simulink model "TP1_Simulink"  (R2021a)
settings: Solver=VariableStepAuto  StartTime=0.0  StopTime=3000  RelTol=1e-3
values from neighbouring files (symbols this model uses):
  A_sim = double(subs(As,{x,u},{x_e,u_e}))    [TPI_Matlab.m]    (also in tp1.m)
  B_sim = double(subs(Bs,{x,u},{x_e,u_e}))    [TPI_Matlab.m]    (also in tp1.m)
  C_sim = double(subs(Cs,{x,u},{x_e,u_e}))    [TPI_Matlab.m]    (also in tp1.m)
  D_sim = double(subs(Ds,{x,u},{x_e,u_e}))    [TPI_Matlab.m]    (also in tp1.m)
  h_e = 0.45    [TPI_Matlab.m]    (also in tp1.m)
  Q_i = 8e-3/60    (= 0.000133333333333)    [TPI_Matlab.m]    (also in ej1.m; tp1.m)
  u_e = Q_i/(pi * d^2 * sqrt(2*G*x_e)/4)    [TPI_Matlab.m]    (also in ej1.m = Q_i./(pi * d^2 * sqrt(2*G*x_e)/4); tp1.m)
  x_e = 0.45    [TPI_Matlab.m]    (also in ej1.m = (0.1:0.1:0.8); tp1.m)
libraries: cstblocks x4
settings Model: Creator=Cristian  LastModifiedBy=nnobi

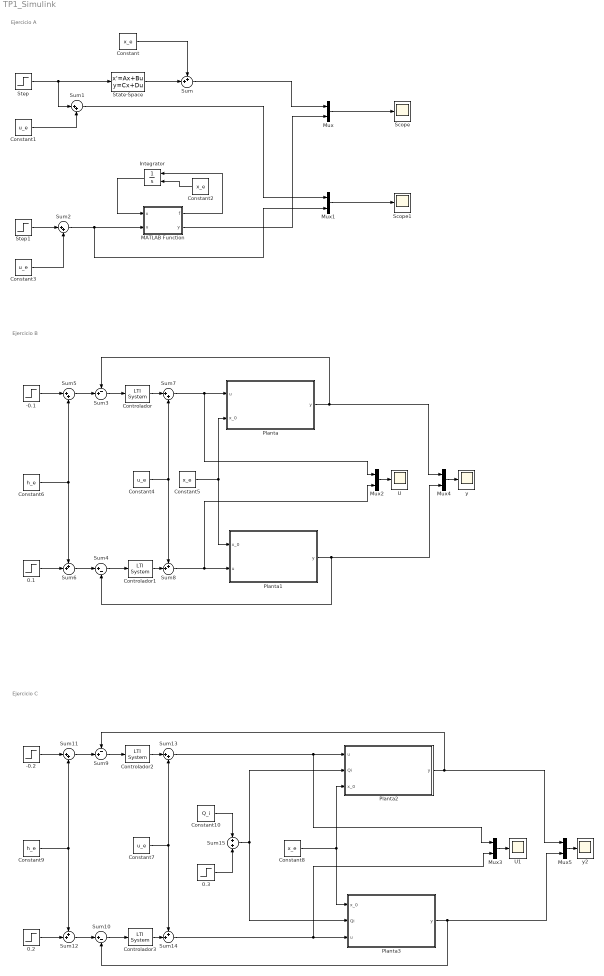
== system TP1_Simulink ==
  note: Ejercicio B
  note: Ejercicio A
  note: Ejercicio C
  -0.1 : Step  Time=60  After=-0.1  SampleTime=0
  -0.2 : Step  Time=60  After=-0.1  SampleTime=0
  0.1 : Step  Time=60  After=0.1  SampleTime=0
  0.2 : Step  Time=60  After=0.1  SampleTime=0
  0.3 : Step  Time=1000  After=-0.1*Q_i  SampleTime=0
  Constant{,2,5,8} (4 alike) : Constant  Value=x_e
  Constant{1,3..4,7} (4 alike) : Constant  Value=u_e
  Constant10 : Constant  Value=Q_i
  Constant6 : Constant  Value=h_e
  Constant9 : Constant  Value=h_e
  Controlador{,1..3} (4 alike) : cstblocks/LTI System  sys=C  IC=[]
  Integrator : Integrator  InitialConditionSource=external
  MATLAB Function : MATLAB Function  TreatAsAtomicUnit=on
  Mux{,1..5} (6 alike) : Mux  Inputs=2
  Planta : Subsystem
  Planta1 : Subsystem
  Planta2 : Subsystem
  Planta3 : Subsystem
  Scope : Scope
  Scope1 : Scope
  State-Space : StateSpace  A=A_sim  B=B_sim  C=C_sim  D=D_sim  InitialCondition=0
  Step : Step  Time=60  After=0.1*u_e  SampleTime=0
  Step1 : Step  Time=60  After=0.1*u_e  SampleTime=0
  Sum{,6,8,12,14} (5 alike) : Sum  Inputs=++|
  Sum{1..2,5,7,11,13} (6 alike) : Sum  Inputs=|++
  Sum10 : Sum  Inputs=|+-
  Sum15 : Sum
  Sum3 : Sum  Inputs=-+|
  Sum4 : Sum  Inputs=|+-
  Sum9 : Sum  Inputs=-+|
  U : Scope
  U1 : Scope
  y : Scope
  y2 : Scope
  wires:
  Step/1 -> Sum1/1, State-Space/1
  State-Space/1 -> Sum/2
  Constant/1 -> Sum/1
  Constant1/1 -> Sum1/2
  Step1/1 -> Sum2/1
  Constant3/1 -> Sum2/2
  Constant2/1 -> Integrator/2
  Sum2/1 -> Mux1/2, MATLAB Function/2(u)
  Integrator/1 -> MATLAB Function/1(x)
  MATLAB Function/1(f) -> Integrator/1
  Mux/1 -> Scope/1
  Sum/1 -> Mux/1
  MATLAB Function/2(y) -> Mux/2
  Sum1/1 -> Mux1/1
  Mux1/1 -> Scope1/1
  Controlador/1 -> Sum7/1
  Sum3/1 -> Controlador/1
  Planta/1(y) -> Mux4/1, Sum3/1
  Constant5/1 -> Planta1/1(x_0), Planta/2(x_0)
  Planta1/1(y) -> Mux4/2, Sum4/2
  Sum4/1 -> Controlador1/1
  Mux2/1 -> U/1
  -0.1/1 -> Sum5/1
  0.1/1 -> Sum6/2
  Constant6/1 -> Sum5/2, Sum6/1
  Sum6/1 -> Sum4/1
  Sum5/1 -> Sum3/2
  Sum7/1 -> Mux2/1, Planta/1(u)
  Controlador1/1 -> Sum8/2
  Sum8/1 -> Mux2/2, Planta1/2(u)
  Constant4/1 -> Sum7/2, Sum8/1
  Sum10/1 -> Controlador3/1
  Planta3/1(y) -> Mux5/2, Sum10/2
  Sum12/1 -> Sum10/1
  Constant9/1 -> Sum11/2, Sum12/1
  Constant7/1 -> Sum13/2, Sum14/1
  Controlador2/1 -> Sum13/1
  Mux3/1 -> U1/1
  Sum11/1 -> Sum9/2
  -0.2/1 -> Sum11/1
  Sum9/1 -> Controlador2/1
  Sum14/1 -> Mux3/2, Planta3/3(u)
  0.2/1 -> Sum12/2
  Sum13/1 -> Mux3/1, Planta2/1(u)
  Constant8/1 -> Planta2/3(x_0), Planta3/1(x_0)
  Controlador3/1 -> Sum14/2
  0.3/1 -> Sum15/2
  Constant10/1 -> Sum15/1
  Sum15/1 -> Planta3/2(Qi), Planta2/2(Qi)
  Mux4/1 -> y/1
  Mux5/1 -> y2/1
  Planta2/1(y) -> Sum9/1, Mux5/1

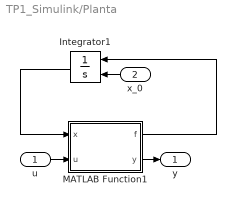
== system TP1_Simulink/Planta ==
  u : Inport
  x_0 : Inport  Port=2
  Integrator1 : Integrator  InitialConditionSource=external
  MATLAB Function1 : MATLAB Function  TreatAsAtomicUnit=on
  y : Outport
  wires:
  MATLAB Function1/1(f) -> Integrator1/1
  Integrator1/1 -> MATLAB Function1/1(x)
  MATLAB Function1/2(y) -> y/1
  u/1 -> MATLAB Function1/2(u)
  x_0/1 -> Integrator1/2

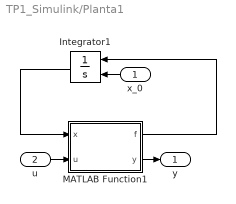
== system TP1_Simulink/Planta1 ==
  x_0 : Inport
  u : Inport  Port=2
  Integrator1 : Integrator  InitialConditionSource=external
  MATLAB Function1 : MATLAB Function  TreatAsAtomicUnit=on
  y : Outport
  wires:
  MATLAB Function1/1(f) -> Integrator1/1
  Integrator1/1 -> MATLAB Function1/1(x)
  MATLAB Function1/2(y) -> y/1
  u/1 -> MATLAB Function1/2(u)
  x_0/1 -> Integrator1/2

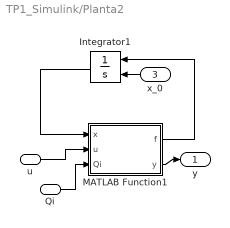
== system TP1_Simulink/Planta2 ==
  u : Inport
  Qi : Inport  Port=2
  x_0 : Inport  Port=3
  Integrator1 : Integrator  InitialConditionSource=external
  MATLAB Function1 : MATLAB Function  TreatAsAtomicUnit=on
  y : Outport
  wires:
  MATLAB Function1/1(f) -> Integrator1/1
  Integrator1/1 -> MATLAB Function1/1(x)
  MATLAB Function1/2(y) -> y/1
  u/1 -> MATLAB Function1/2(u)
  x_0/1 -> Integrator1/2
  Qi/1 -> MATLAB Function1/3(Qi)

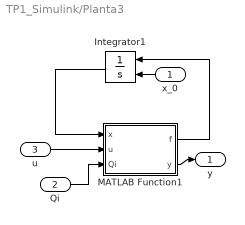
== system TP1_Simulink/Planta3 ==
  x_0 : Inport
  Qi : Inport  Port=2
  u : Inport  Port=3
  Integrator1 : Integrator  InitialConditionSource=external
  MATLAB Function1 : MATLAB Function  TreatAsAtomicUnit=on
  y : Outport
  wires:
  MATLAB Function1/1(f) -> Integrator1/1
  Integrator1/1 -> MATLAB Function1/1(x)
  MATLAB Function1/2(y) -> y/1
  u/1 -> MATLAB Function1/2(u)
  x_0/1 -> Integrator1/2
  Qi/1 -> MATLAB Function1/3(Qi)

== matlab function TP1_Simulink/Planta/MATLAB Function1 ==
  data: x input; f output; u input; y output
function [f,y] = fcn(x,u)
G = 9.8;

a_max = 0.4;
h_max = 0.9;
b = 0.1;
d = 0.01065;
Q_i = 8e-3/60;

m = (a_max - b)/h_max;

f = (Q_i - pi * d^2 * sqrt(2*G*x)*u/4 )/(m^2 * x^2 + 2*b*m*x + b^2);

y = x;

== matlab function TP1_Simulink/MATLAB Function ==
  data: x input; f output; u input; y output
function [f,y] = fcn(x,u)
G = 9.8;

a_max = 0.4;
h_max = 0.9;
b = 0.1;
d = 0.01065;
Q_i = 8e-3/60;

m = (a_max - b)/h_max;

f = (Q_i - pi * d^2 * sqrt(2*G*x)*u/4 )/(m^2 * x^2 + 2*b*m*x + b^2);

y = x;

== matlab function TP1_Simulink/Planta1/MATLAB Function1 ==
  data: x input; f output; u input; y output
function [f,y] = fcn(x,u)
G = 9.8;

a_max = 0.4;
h_max = 0.9;
b = 0.1;
d = 0.01065;
Q_i = 8e-3/60;

m = (a_max - b)/h_max;

f = (Q_i - pi * d^2 * sqrt(2*G*x)*u/4 )/(m^2 * x^2 + 2*b*m*x + b^2);

y = x;

== matlab function TP1_Simulink/Planta2/MATLAB Function1 ==
  data: x input; f output; u input; y output; Qi input
function [f,y] = fcn(x,u,Qi)
G = 9.8;

a_max = 0.4;
h_max = 0.9;
b = 0.1;
d = 0.01065;

m = (a_max - b)/h_max;

f = (Qi - pi * d^2 * sqrt(2*G*x)*u/4 )/(m^2 * x^2 + 2*b*m*x + b^2);

y = x;

== matlab function TP1_Simulink/Planta3/MATLAB Function1 ==
  data: x input; f output; u input; y output; Qi input
function [f,y] = fcn(x,u,Qi)
G = 9.8;

a_max = 0.4;
h_max = 0.9;
b = 0.1;
d = 0.01065;

m = (a_max - b)/h_max;

f = (Qi - pi * d^2 * sqrt(2*G*x)*u/4 )/(m^2 * x^2 + 2*b*m*x + b^2);

y = x;
